simulink model "fin_pro_identi_sim"  (R2023b)
settings: Solver=ode4  StartTime=0.0  StopTime=20  FixedStep=0.005  RelTol=1e-3
values from neighbouring files (symbols this model uses):
  hat_A = ([params(1), params(2); params(3), params(4)])    [fin_pro_identi_mat.m]
  hat_B = ([params(5), 0; 0, params(6)])    [fin_pro_identi_mat.m]
  hat_f1 = params(7)    [fin_pro_identi_mat.m]
  hat_f2 = params(8)    [fin_pro_identi_mat.m]
settings Model: Creator=wook9  LastModifiedBy=wook9

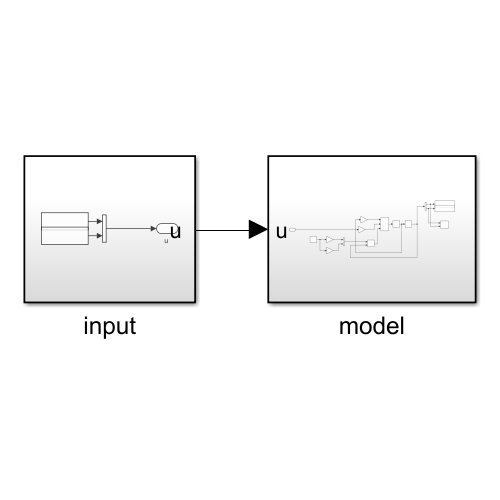
[thumbnail: Simulink's stored preview of the top-level diagram]
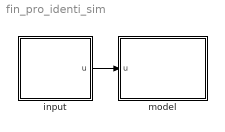
== system fin_pro_identi_sim ==
  input : Subsystem
  model : Subsystem
  wires:
  input/1("u ") -> model/1(u)

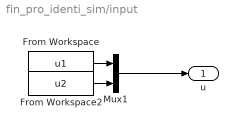
== system fin_pro_identi_sim/input ==
  From Workspace : FromWorkspace  VariableName=u1
  From Workspace2 : FromWorkspace  VariableName=u2
  Mux1 : Mux  Inputs=2
  "u " : Outport
  wires:
  From Workspace/1 -> Mux1/1
  From Workspace2/1 -> Mux1/2
  Mux1/1 -> "u "/1

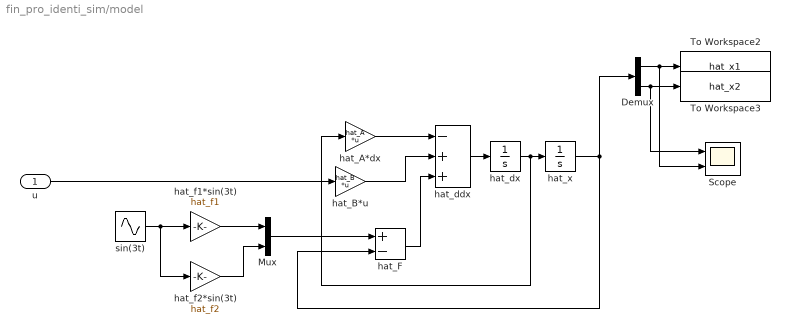
== system fin_pro_identi_sim/model ==
  u : Inport
  Demux : Demux  Outputs=2
  Mux : Mux  Inputs=2
  Scope : Scope  NumInputPorts=2
  To Workspace2 : ToWorkspace  VariableName=hat_x1  SampleTime=-1
      settings: Save2DSignal=2-D array (concatenate along first dimension)
  To Workspace3 : ToWorkspace  VariableName=hat_x2  SampleTime=-1
      settings: Save2DSignal=2-D array (concatenate along first dimension)
  hat_A*dx : Gain  Gain=hat_A  Multiplication=Matrix(K*u) (u vector)
  hat_B*u : Gain  Gain=hat_B  Multiplication=Matrix(K*u) (u vector)
  hat_F : Sum  Inputs=+-
  hat_ddx : Sum  Inputs=-++
  hat_dx : Integrator  InitialCondition=[0; 0]
  hat_f1*sin(3t) : Gain  Gain=hat_f1
  hat_f2*sin(3t) : Gain  Gain=hat_f2
  hat_x : Integrator  InitialCondition=[0; 0]
  sin(3t) : Sin  Frequency=3  SampleTime=0
  wires:
  hat_x/1 -> Demux/1, hat_F/2
  hat_f1*sin(3t)/1 -> Mux/1
  hat_dx/1 -> hat_A*dx/1, hat_x/1
  hat_f2*sin(3t)/1 -> Mux/2
  Demux/1 -> Scope/2, To Workspace2/1
  hat_ddx/1 -> hat_dx/1
  Demux/2 -> Scope/1, To Workspace3/1
  hat_A*dx/1 -> hat_ddx/1
  hat_B*u/1 -> hat_ddx/2
  Mux/1 -> hat_F/1
  sin(3t)/1 -> hat_f1*sin(3t)/1, hat_f2*sin(3t)/1
  hat_F/1 -> hat_ddx/3
  u/1 -> hat_B*u/1
